simulink model "ReadWaveform"  (R2020a)
settings: Solver=FixedStepAuto  StartTime=0.0  StopTime=10.0  FixedStep=1e-3  RelTol=1e-3  EnableMultiTasking=on
undefined symbols (not defined in the file): A0, A1, D13, PTB2, PTB3, PTD1
libraries: frdmk64flib x3, etargetslib x3
settings Model: ExtModeTrigDuration=5  Creator=WinnieTrandinh  LastModifiedBy=WinnieTrandinh
settings OptimizationCC: EnhancedBackFolding=on  PassReuseOutputArgsAs=Individual arguments  ZeroExternalMemoryAtStartup=off  ZeroInternalMemoryAtStartup=off  MaxStackSize=64  OptimizeBlockOrder=speed  DifferentSizesBufferReuse=on  OptimizationCustomize=off  EfficientTunableParamExpr=on
settings DebuggingCC: ParameterTunabilityLossMsg=error
settings HardwareCC: ProdBitPerPointer=32  ProdBitPerSizeT=32  ProdBitPerPtrDiffT=32  ProdLargestAtomicInteger=Long  ProdLargestAtomicFloat=Double  ProdWordSize=32  ProdHWDeviceType=ARM Compatible->ARM Cortex
settings SFSimCC: MATLABDynamicMemAlloc=off
settings RTWCC: SystemTargetFile=ert.tlc  HardwareBoard=NXP FRDM-K64F  TemplateMakefile=ert_default_tmf  Toolchain=GNU Tools for ARM Embedded Processors
settings CodeAppCC: ForceParamTrailComments=on  IgnoreCustomStorageClasses=off  OperatorAnnotations=on  SimulinkDataObjDesc=on  SFDataObjDesc=on  InsertBlockDesc=on

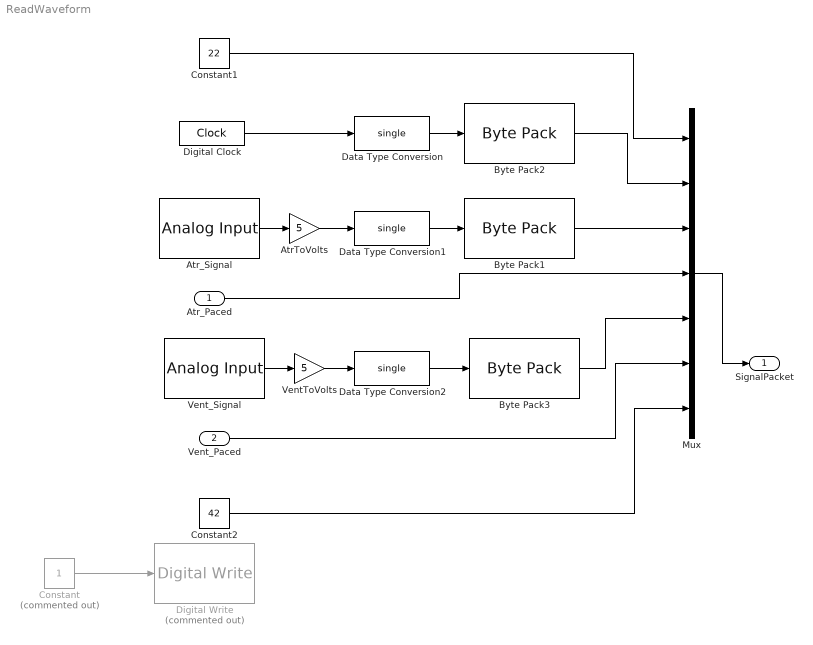
== system ReadWaveform ==
  Atr_Paced : Inport  OutDataTypeStr=uint8
  Vent_Paced : Inport  Port=2  OutDataTypeStr=uint8
  AtrToVolts : Gain  Gain=5
  Atr_Signal : frdmk64flib/Analog Input  Whichpin=PTB2 (A0)  SampleTime=-1
  Byte Pack1 : etargetslib/Byte Pack  datatypes={'single'}  byteAlign=1
  Byte Pack2 : etargetslib/Byte Pack  datatypes={'single'}  byteAlign=1
  Byte Pack3 : etargetslib/Byte Pack  datatypes={'single'}  byteAlign=1
  Constant : Constant  Commented=on
  Constant1 : Constant  Value=22  OutDataTypeStr=uint8
  Constant2 : Constant  Value=42  OutDataTypeStr=uint8
  Data Type Conversion : DataTypeConversion  OutDataTypeStr=single
  Data Type Conversion1 : DataTypeConversion  OutDataTypeStr=single
  Data Type Conversion2 : DataTypeConversion  OutDataTypeStr=single
  Digital Clock : DigitalClock  SampleTime=0.001
  Digital Write : frdmk64flib/Digital Write  Commented=on  Whichpin=PTD1 (D13)
  Mux : Mux  Inputs=7
  VentToVolts : Gain  Gain=5
  Vent_Signal : frdmk64flib/Analog Input  Whichpin=PTB3 (A1)  SampleTime=-1
  SignalPacket : Outport
  wires:
  Atr_Signal/1 -> AtrToVolts/1
  Vent_Signal/1 -> VentToVolts/1
  AtrToVolts/1 -> Data Type Conversion1/1
  VentToVolts/1 -> Data Type Conversion2/1
  Constant/1 -> Digital Write/1
  Mux/1 -> SignalPacket/1
  Constant1/1 -> Mux/1
  Byte Pack1/1 -> Mux/3
  Digital Clock/1 -> Data Type Conversion/1
  Byte Pack2/1 -> Mux/2
  Data Type Conversion/1 -> Byte Pack2/1
  Data Type Conversion1/1 -> Byte Pack1/1
  Data Type Conversion2/1 -> Byte Pack3/1
  Constant2/1 -> Mux/7
  Atr_Paced/1 -> Mux/4
  Vent_Paced/1 -> Mux/6
  Byte Pack3/1 -> Mux/5
